simulink model "lab4_part2_question3"  (R2023a)
settings: Solver=VariableStepAuto  StartTime=0.0  StopTime=10.0  RelTol=1e-3
libraries: dspsnks4 x1, dspvision x1
settings Model: Creator=ma_kaba  LastModifiedBy=ma_kaba

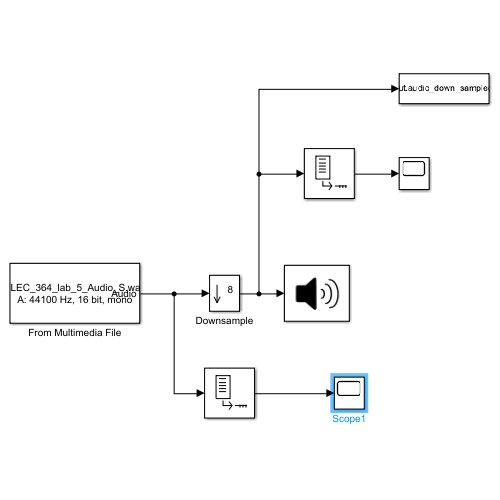
[thumbnail: Simulink's stored preview of the top-level diagram]
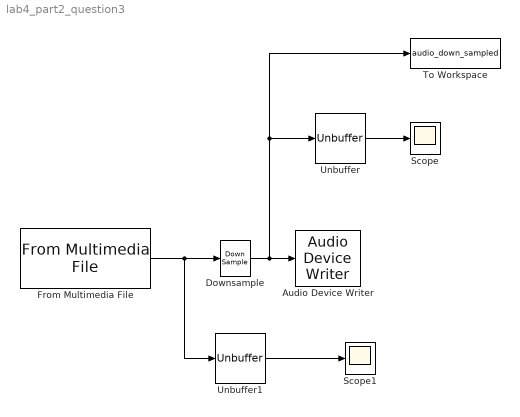
== system lab4_part2_question3 ==
  Audio Device Writer : dspsnks4/Audio Device Writer  Driver=DirectSound  Device=Default  InheritSampleRate=on  SampleRate=44100  BitDepth=16-bit integer  BufferSize=4096  NumBuffers=10  DefaultOutputChannelMapping=on  OutputChannelMapping=1:2  OutputNumUnderrunSamples=off  DriverIdx=1  DeviceWarnFlag=''
  Downsample : DownSample  N=8  RateOptions=Allow multirate processing
  From Multimedia File : dspvision/From Multimedia File  inputFilename=G:\My Documents\MATLAB\ELEC_364_lab_5_Audio_S.wav  readRange=[1 Inf]  loop=on  numPlays=inf  outputStreams=Audio only  videoDataType=single  audioDataType=double  inheritSampleTime=on  userDefinedSampleTime=1/30  noAudioOutput=off  isIntensityVideo=off  fourcc=RGB  colorVideoFormat=Separate color signals  outputEOF=off  dataOrg=Column-major  audioFrameSize=1024  computeAudioFrameSize=off  outSamplingMode=Sample based
      settings: LibrarySourceBlock=dspsrcs4/From Multimedia File
  Scope : Scope
  Scope1 : Scope
  To Workspace : ToWorkspace  VariableName=audio_down_sampled  SaveFormat=Timeseries  SampleTime=-1
  Unbuffer : Unbuffer
  Unbuffer1 : Unbuffer
  wires:
  Downsample/1 -> To Workspace/1, Unbuffer/1, Audio Device Writer/1
  Unbuffer/1 -> Scope/1
  From Multimedia File/1 -> Unbuffer1/1, Downsample/1
  Unbuffer1/1 -> Scope1/1
